simulink library "MainLibrary"  (R2020a)
settings: Solver=VariableStepAuto  StartTime=0.0  StopTime=10.0  RelTol=1e-3
settings Model: Creator=AlexC  LastModifiedBy=AlexC
settings DataIOCC: ReturnWorkspaceOutputs=off
settings DebuggingCC: ArithmeticOperatorsInVariantConditions=warning
settings SFSimCC: SimUseLocalCustomCode=off  CustomCodeUndefinedFunction=UseInterfaceOnly
settings RTWCC: RTWUseLocalCustomCode=off

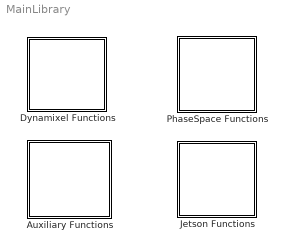
== system MainLibrary ==
  Auxiliary Functions : Subsystem
  Dynamixel Functions : Subsystem
  Jetson Functions : Subsystem
  PhaseSpace Functions : Subsystem

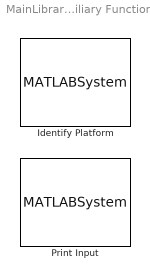
== system MainLibrary/Auxiliary Functions ==
  Identify Platform : MATLABSystem  System=IdentifyPlatform  SampleTime=0.01
      mask Type: IdentifyPlatform
      mask Display:
      | disp('IdentifyPlatform');
      | port_label('output',1,'y');
  Print Input : MATLABSystem  System=Debugging
      mask Type: Debugging
      mask Display:
      | disp('Debugging');
      | port_label('input',1,'u');

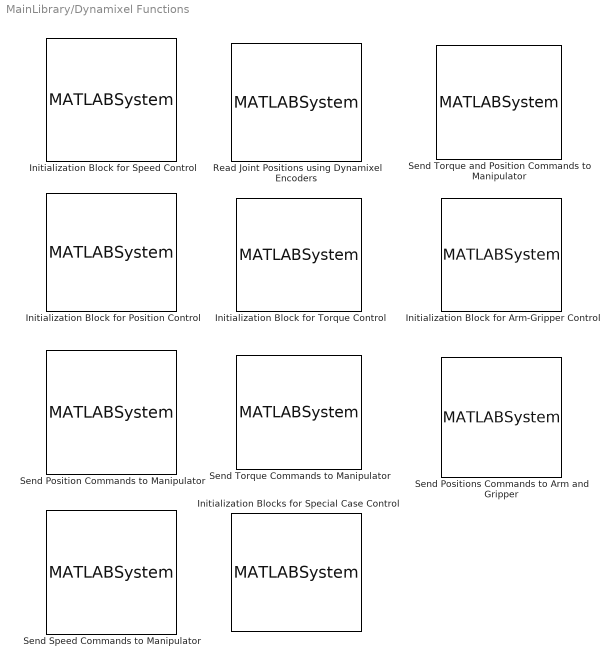
== system MainLibrary/Dynamixel Functions ==
  Initialization Block for Arm-Gripper Control : MATLABSystem  System=InitializeForArmGripper  P_GAIN_ARM=400  I_GAIN_ARM=0  D_GAIN_ARM=200  P_GAIN_PROX=400  I_GAIN_PROX=0  D_GAIN_PROX=200  P_GAIN_DIST=400  I_GAIN_DIST=0  D_GAIN_DIST=200  MAX_POSITION_ARM=3072  MIN_POSITION_ARM=1024  MAX_POSITION_PROX=3072  MIN_POSITION_PROX=1024  MAX_POSITION_DIST=3072  MIN_POSITION_DIST=1024  VELOCITY_LIMIT_ARM=0  VELOCITY_LIMIT_GRIP=0  MAX_CURRENT_GRIP=1000
      mask Type: InitializeForArmGripper
      mask Display: disp('InitializeForArmGripper');
  Initialization Block for Position Control : MATLABSystem  System=InitializeForPosition  P_GAIN=400  I_GAIN=0  D_GAIN=200  MAX_POSITION=4095  MIN_POSITION=0  VELOCITY_LIMIT=380
      mask Type: InitializeForPosition
      mask Display: disp('InitializeForPosition');
  Initialization Block for Speed Control : MATLABSystem  System=InitializeForSpeed  P_GAIN=100  I_GAIN=1920  VELOCITY_LIMIT=1023
      mask Type: InitializeForSpeed
      mask Display: disp('InitializeForSpeed');
  Initialization Block for Torque Control : MATLABSystem  System=InitializeForTorque  CURRENT_LIMIT=850
      mask Type: InitializeForTorque
      mask Display: disp('InitializeForTorque');
  Initialization Blocks for Special Case Control : MATLABSystem  System=InitializeForSpecial  CURRENT_LIMIT=850  P_GAIN=400  I_GAIN=0  D_GAIN=200  MAX_POSITION=3072  MIN_POSITION=1024  VELOCITY_LIMIT=0
      mask Type: InitializeForSpecial
      mask Display: disp('InitializeForSpecial');
  Read Joint Positions using Dynamixel Encoders : MATLABSystem  System=ReadArm_Position  SampleTime=0.05
      mask Type: ReadArm_Position
      mask Display:
      | disp('ReadArm_Position');
      | port_label('output',1,'y1');
      | port_label('output',2,'y2');
      | port_label('output',3,'y3');
  Send Position Commands to Manipulator : MATLABSystem  System=MoveArm_Position
      mask Type: MoveArm_Position
      mask Display:
      | disp('MoveArm_Position');
      | port_label('input',1,'u1');
      | port_label('input',2,'u2');
      | port_label('input',3,'u3');
  Send Positions Commands to Arm and Gripper : MATLABSystem  System=MoveArmGripper_Position
      mask Type: MoveArmGripper_Position
      mask Display:
      | disp('MoveArmGripper_Position');
      | port_label('input',1,'u1');
      | port_label('input',2,'u2');
      | port_label('input',3,'u3');
      | port_label('input',4,'uL1');
      | port_label('input',5,'uR1');
      | port_label('input',6,'uL2');
      | port_label('input',7,'uR2');
  Send Speed Commands to Manipulator : MATLABSystem  System=MoveArm_Speed
      mask Type: MoveArm_Speed
      mask Display:
      | disp('MoveArm_Speed');
      | port_label('input',1,'u1');
      | port_label('input',2,'u2');
      | port_label('input',3,'u3');
  Send Torque Commands to Manipulator : MATLABSystem  System=MoveArm_Torque
      mask Type: MoveArm_Torque
      mask Display:
      | disp('MoveArm_Torque');
      | port_label('input',1,'u1');
      | port_label('input',2,'u2');
      | port_label('input',3,'u3');
  Send Torque and Position Commands to Manipulator : MATLABSystem  System=MoveArm_Special
      mask Type: MoveArm_Special
      mask Display:
      | disp('MoveArm_Special');
      | port_label('input',1,'u1');
      | port_label('input',2,'u2');
      | port_label('input',3,'u3');

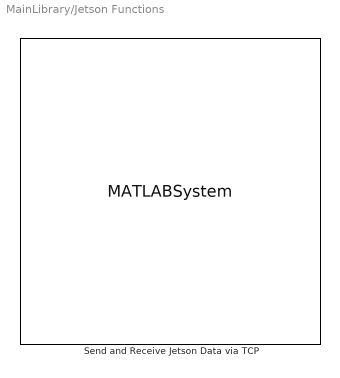
== system MainLibrary/Jetson Functions ==
  Send and Receive Jetson Data via TCP : MATLABSystem  System=guidance_server
      mask Type: guidance_server
      mask Display: disp('guidance_server');
  wires:
  ? -> Send and Receive Jetson Data via TCP/1

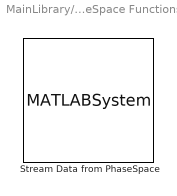
== system MainLibrary/PhaseSpace Functions ==
  Stream Data from PhaseSpace : MATLABSystem  System=PhaseSpace_ALL  platformSelection=1
      mask Type: PhaseSpace_ALL
      mask Display:
      | disp('Stream_PS_ALL');
      | port_label('output',1,'y');
